simulink model "DroneController"  (R2024b)
settings: Solver=VariableStepAuto  StartTime=0.0  StopTime=30  RelTol=1e-3
undefined symbols (not defined in the file or in its folder): Sim3dSensor
libraries: shared6dof x1, sharedtransform x1, sim3dcameralib x1, sim3dlib x1, uavsim3dlib x1, uavutilslib x1
settings Model: Creator=Rayhaan T  LastModifiedBy=Rayhaan T

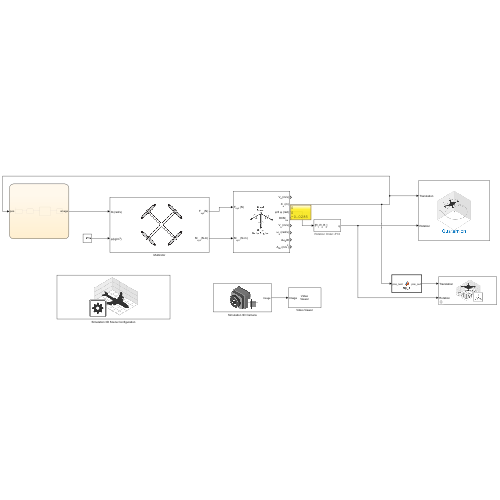
[thumbnail: Simulink's stored preview of the top-level diagram]
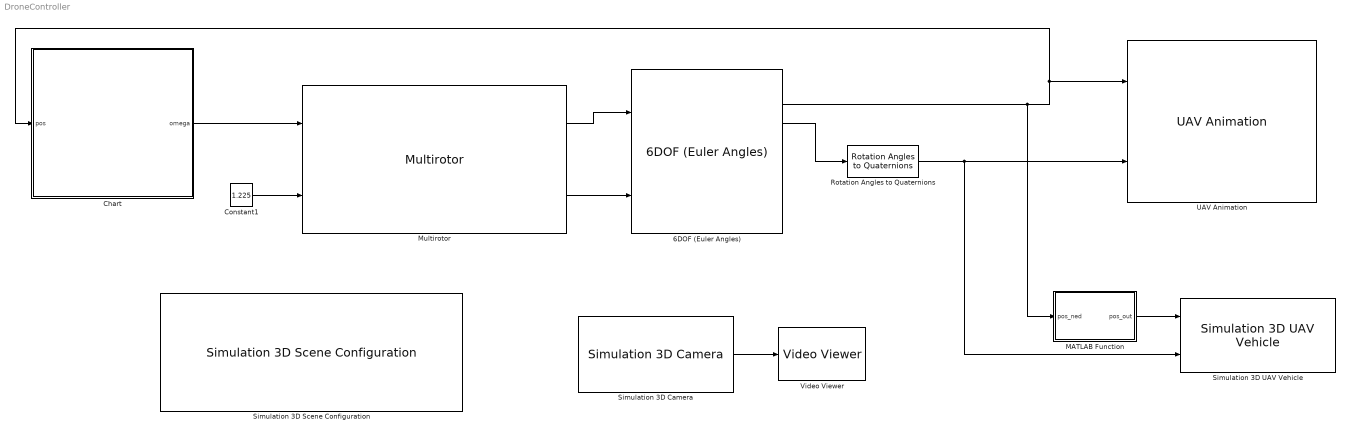
== system DroneController ==
  6DOF (Euler Angles) : shared6dof/6DOF (Euler Angles)  units=Metric (MKS)  mtype=Fixed  rep=Euler Angles  xme_0=[0 0 0]  Vm_0=[0 0 0]  eul_0=[0 0 0]  pm_0=[0 0 0]  mass_0=0.5  mass_e=0.5  mass_f=2.0  inertia=eye(3)  inertia_e=eye(3)  inertia_f=2*eye(3)  k_quat=1.0  vre_flag=on  abi_flag=off  aMode=0  xme_statename=''  Vm_statename=''  eul_statename=''  quat_statename=''  pm_statename=''  mass_statename=''
  Chart : Stateflow chart  TreatAsAtomicUnit=on
  Constant1 : Constant  Value=1.225
  MATLAB Function : MATLAB Function  TreatAsAtomicUnit=on
  Multirotor : Multirotor
  Rotation Angles to Quaternions : sharedtransform/Rotation Angles to Quaternions  rotationOrder=ZYX  aMode=aMode
  Simulation 3D Camera : sim3dcameralib/Simulation 3D Camera  Priority=1  sensorTag=Sim3dSensor�  sensorId=1  sensorName=Sim3dSensor�  vehTagList={'Scene Origin';'SimulinkVehicle1'}  vehTag=SimulinkVehicle1  mountLoc=Origin  offsetFlag=on  tmountOffset=[0, 0, 0.1]  extTmount=off  rmountOffset=[0, 90, 0]  extRmount=off  FocalLength=[320, 320]  OpticalCenter=[160, 120]  ImageSize=[240, 320]  RadialDistortion=[0, 0]  TangentialDistortion=[0, 0]  SensorSkew=0  DepthOutportEnabled=off  SemanticOutportEnabled=off  TransformOutportEnabled=off  SampleTime=0.1  mountPoint=[0 0 0.1]  mountOrientation=[0 -90 0]  aMode=4  ID=1
      settings: LibrarySourceBlock=uavsim3dlib/Simulation 3D Camera
  Simulation 3D Scene Configuration : sim3dlib/Simulation 3D Scene Configuration  Priority=0  ProjectFormat=Default Scenes  SceneDesc=Airport  ProjectName=D:\matlab_dnd\toolbox\shared\sim3d_projects\automotive_project_windows\UE\WindowsNoEditor\VehicleSimulation.exe  ScenePath=/Game/Maps/HwStrght  EnableOpenDRIVE=off  vehTagList={'Custom';'Scene Origin';'SimulinkVehicle1'}  vehTag=Scene Origin  FreeCameraInitialTranslation=[-6, 0, 2]  FreeCameraDefaultInitialTranslation=[-6, 0, 2]  FreeCameraInitialRotation=[0, -15, 0]  FreeCameraDefaultInitialRotation=[0, -15, 0]  OpVisEn=off  Ts=.01  EnableWindow=on  EnableRemoteAccess=off  EnableWeather=off  SunAzimuth=90  SunAltitude=40.0  EnableGeospatialSun=off  Latitude=0  Longitude=0  Date=2023-01-01  Time=10:30:00  GeoTimeZone=-5.0  SunDaylightSaving=off  wind=1  clouds=10  EnableVolumetricClouds=off  CloudCoverage=0  CloudAltitude=6  fog=0  rain=0  RaindropsEffect=off  SnowDensity=0  EnableGeospatial=off  UseTrueOrigin=off  OriginHeight=200  OriginLatitude=40.744652  OriginLongitude=-73.988864  MapStyle=Aerial  AdditionalAssetIDs=[]  UseAdvancedSunSky=off  SolarTime=11  TimeZone=-5  Day=21  Month=9  Year=2022  UseDaylightSavingTime=on  DSTStartDay=10  DSTStartMonth=3  DSTEndDay=3  DSTEndMonth=11  DSTSwitchHour=2  sensorTag=MainCamera1  sensorId=1  sensorName=MainCamera1  mountLoc=Origin  offsetFlag=off  tmountOffset=[0, 0, 0]  rmountOffset=[0, 0, 0]  HorizontalResolution=1280  VerticalResolution=720  HorizontalFOV=60  mountPoint=[0 0 0]  mountOrientation=[0 0 0]  aMode=0  ID=1  GeoTrigger=Inactive
      settings: LibrarySourceBlock=aerolibsim3d/Simulation 3D Scene Configuration
  Simulation 3D UAV Vehicle : uavsim3dlib/Simulation 3D UAV Vehicle  Priority=-1  Mesh=Quadrotor  MeshPath=/MathWorksUAVContent/UAVs/HexaRotorUAV/HexaRotor.HexaRotor  Color=Black  ActorName=SimulinkVehicle1  UseGlobalFrame=off  InitialTranslation=[0 0 0]  InitialRotation=[0 0 0]  InitialTranslationGlobal=[0 0 0]  InitialGeoOrigin=[0 0 0]  InitialRotationGlobal=[0 0 0]  SampleTime=0.01  ActorType=SimulinkVehicle  ID=1  aMode=4  ActorTag=SimulinkVehicle1
  UAV Animation : uavutilslib/UAV Animation  NumUAV=1  DynamicUAVConfig=off  UAVType=Multirotor  UAVSize=1  UAVColor=[1 0 0]  UAVTrajectoryAlpha=1  InertialZDirection=Down  RotationFormat=Quaternion  DrawMarkers=off  SampleTime=0.01
  Video Viewer : VideoViewer  FigPos=[944.2 581.2 417.6 304]
  wires:
  Constant1/1 -> Multirotor/2
  Multirotor/1 -> 6DOF (Euler Angles)/1
  Multirotor/2 -> 6DOF (Euler Angles)/2
  6DOF (Euler Angles)/2 -> UAV Animation/1, Chart/1(pos), MATLAB Function/1(pos_ned)
  6DOF (Euler Angles)/3 -> Rotation Angles to Quaternions/1
  Chart/1(omega) -> Multirotor/1
  Rotation Angles to Quaternions/1 -> Simulation 3D UAV Vehicle/2, UAV Animation/2
  MATLAB Function/1(pos_out) -> Simulation 3D UAV Vehicle/1
  Simulation 3D Camera/1 -> Video Viewer/1

== matlab function DroneController/MATLAB Function ==
  data: pos_ned input; pos_out output
function pos_out = flip_z(pos_ned)
    % NED to 3D Viewer coordinate conversion
    % NED:      X=North, Y=East,  Z=Down
    % 3D Viewer: X=East,  Y=North, Z=Up
    pos_out = [pos_ned(2), pos_ned(1), -pos_ned(3)];
end

== stateflow chart DroneController/Chart ==
  state FOLLOW_LINE
    en: active_state = 2;
    du: % Calculate drift from line (Y should always be 0)
    drift = pos(2);
    % Correct left/right based on drift
    omega_left  = 140 + (5 * drift);
    omega_right = 140 - (5 * drift);
    omega = [omega_left, 140, 140, omega_right];
    % Move forward until X reaches 15m
    if pos(1) >= 15.0
    active_state = 3;
    end
  state TAKEOFF
    en: omega = [140 140 140 140];
    du: if pos(3) <= -2.0
    active_state = 2;
    end
  state LAND
    en: active_state = 3;
    du: omega = [400 400 400 400];
    if pos(3) >= -0.1
    omega = zeros(1,4);
    end
  state IDLE
    en: omega = zeros(1,4);
  (default) -> IDLE
  IDLE -> TAKEOFF : [active_state == 1]
  TAKEOFF -> FOLLOW_LINE : [active_state == 2]
  FOLLOW_LINE -> LAND : [active_state == 3]
  data: pos input double size=[1 3]; omega output double size=[1 4]; active_state local double size=1 =1; drift local; omega_left local; omega_right local
